simulink model "Lab_5_CHE381_220007"  (R2022b)
settings: Solver=VariableStepAuto  StartTime=0.0  StopTime=50  RelTol=1e-3
values from neighbouring files (symbols this model uses):
  Kc = 15    [CHE381_Lab_5_matfile_220007.m]
  tau_d = 2    [CHE381_Lab_5_matfile_220007.m]
  tau_i = 191.822    [CHE381_Lab_5_matfile_220007.m]
settings Model: Creator=Administrator  LastModifiedBy=Administrator

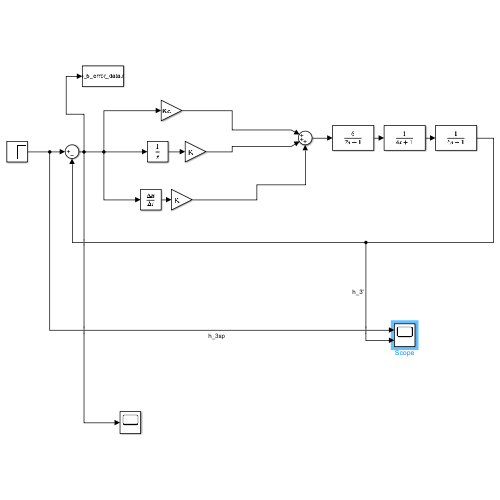
[thumbnail: Simulink's stored preview of the top-level diagram]
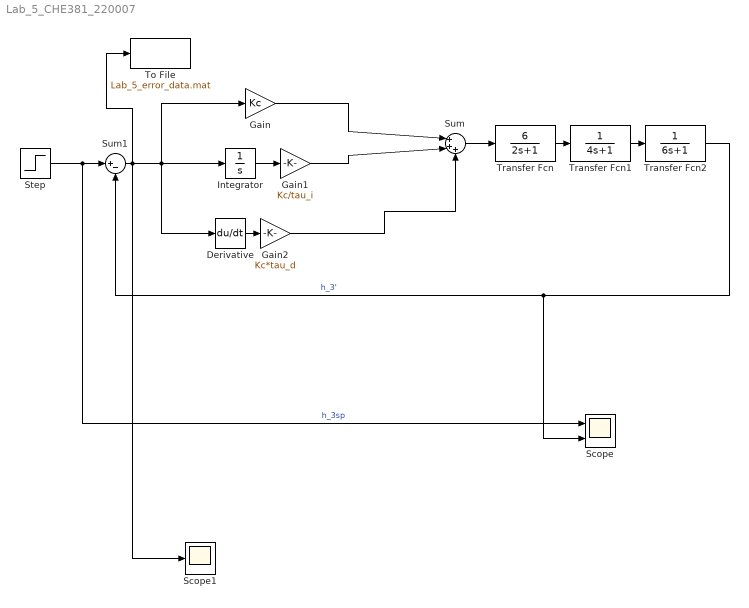
== system Lab_5_CHE381_220007 ==
  Derivative : Derivative
  Gain : Gain  Gain=Kc
  Gain1 : Gain  Gain=Kc/tau_i
  Gain2 : Gain  Gain=Kc*tau_d
  Integrator : Integrator
  Scope : Scope  NumInputPorts=2
  Scope1 : Scope
  Step : Step  Time=0  SampleTime=0
  Sum : Sum  Inputs=|+++
  Sum1 : Sum  Inputs=|+-
  To File : ToFile  Filename=Lab_5_error_data.mat  SampleTime=0.1
  Transfer Fcn : TransferFcn  Numerator=[6]  Denominator=[2 1]
  Transfer Fcn1 : TransferFcn  Denominator=[4 1]
  Transfer Fcn2 : TransferFcn  Denominator=[6 1]
  wires:
  Gain/1 -> Sum/1
  Derivative/1 -> Gain2/1
  Integrator/1 -> Gain1/1
  Gain1/1 -> Sum/2
  Gain2/1 -> Sum/3
  Sum/1 -> Transfer Fcn/1
  Transfer Fcn/1 -> Transfer Fcn1/1
  Transfer Fcn1/1 -> Transfer Fcn2/1
  Transfer Fcn2/1 -> Scope/2, Sum1/2  "h_3'"
  Step/1 -> Scope/1, Sum1/1  "h_3sp"
  Sum1/1 -> To File/1, Scope1/1, Derivative/1, Gain/1, Integrator/1
